simulink subsystem "Maneuver"  (R2021a)
settings: Solver=VariableStepAuto  StartTime=0.0  StopTime=10.0  RelTol=1e-3
undefined symbols (not defined in the file): t0x, t0y, t0z, tfx, tfy, tfz, wx, wy, wz
settings Model: Creator=Laura  LastModifiedBy=Laura

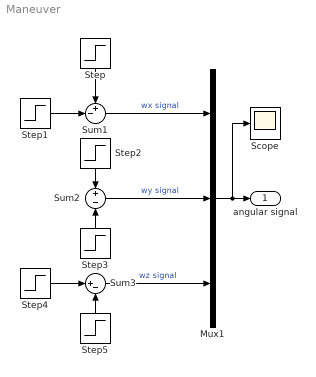
== system Maneuver ==
  Mux1 : Mux  Inputs=3
  Scope : Scope
  Step : Step  Time=t0x  After=wx  SampleTime=0
  Step1 : Step  Time=tfx  After=wx  SampleTime=0
  Step2 : Step  Time=t0y  After=wy  SampleTime=0
  Step3 : Step  Time=tfy  After=wy  SampleTime=0
  Step4 : Step  Time=t0z  After=wz  SampleTime=0
  Step5 : Step  Time=tfz  After=wz  SampleTime=0
  Sum1 : Sum  Inputs=+-|
  Sum2 : Sum  Inputs=+-
  Sum3 : Sum  Inputs=|+-
  angular signal : Outport
  wires:
  Mux1/1 -> Scope/1, angular signal/1
  Step1/1 -> Sum1/2
  Step/1 -> Sum1/1
  Step2/1 -> Sum2/1
  Step3/1 -> Sum2/2
  Sum2/1 -> Mux1/2  "wy signal"
  Step4/1 -> Sum3/1
  Step5/1 -> Sum3/2
  Sum3/1 -> Mux1/3  "wz signal"
  Sum1/1 -> Mux1/1  "wx signal"
